simulink model "testbed"  (R2017b)
settings: Solver=FixedStepAuto  StartTime=0.0  StopTime=inf  FixedStep=0.001  RelTol=1e-3  EnableMultiTasking=on
libraries: xpcethercatlib x22, slrtlib x1
settings Model: xpc_rtwmakecfg_data=_xpcethercatlib_  SimulationMode=external  Creator=motor_testbed  LastModifiedBy=motor_testbed
settings SolverCC: ConcurrentTasks=on  AutoInsertRateTranBlk=on
settings DataIOCC: SaveFormat=StructureWithTime
settings OptimizationCC: BlockReduction=off  OptimizeBlockIOStorage=off  BufferReuse=off  GlobalBufferReuse=off  ExpressionFolding=off  LocalBlockOutputs=off
settings HardwareCC: ProdBitPerPointer=32  ProdBitPerSizeT=32  ProdBitPerPtrDiffT=32  ProdLargestAtomicFloat=None  ProdWordSize=32  ProdLongLongMode=on  ProdHWDeviceType=Generic->32-bit x86 compatible
settings RTWCC: SystemTargetFile=slrt.tlc  TemplateMakefile=slrt_default_tmf  Description=Simulink Real-Time  CodeExecutionProfiling=on  RTWCompilerOptimization=on
settings SimulinkRealTimeCC: SupportVariableSizeSignals=on  RL32LogTETModifier=off  xPCConcurrentTasks=on

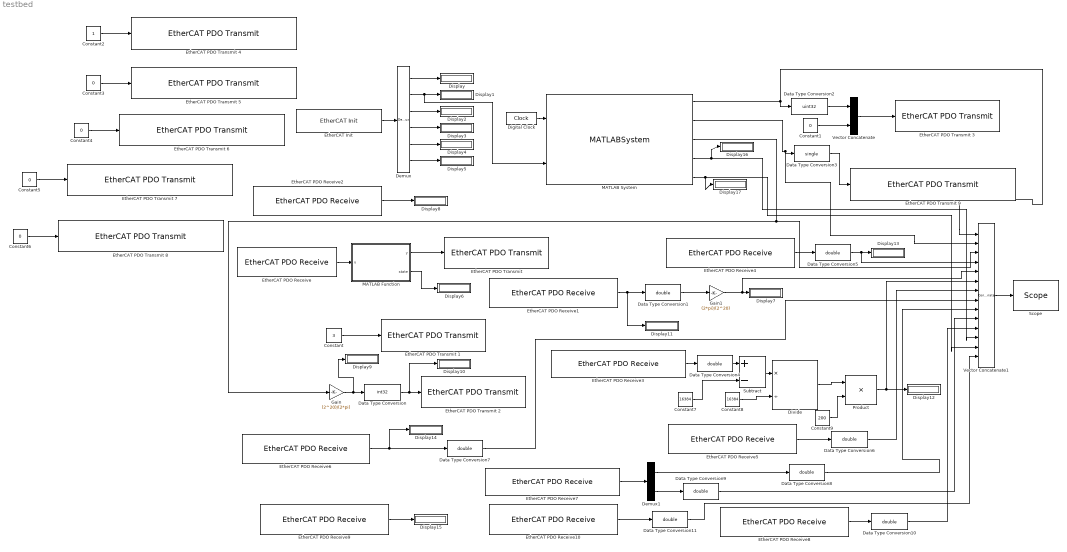
== system testbed ==
  Constant : Constant  Value=3  OutDataTypeStr=int8  SampleTime=0.001
  Constant1 : Constant  Value=0  OutDataTypeStr=uint32  SampleTime=0.001
  Constant2 : Constant  OutDataTypeStr=uint32  SampleTime=0.001
  Constant{3..6} (4 alike) : Constant  Value=0  OutDataTypeStr=single  SampleTime=0.001
  Constant7 : Constant  Value=16384  OutDataTypeStr=double  SampleTime=0.001
  Constant8 : Constant  Value=16384  OutDataTypeStr=double  SampleTime=0.001
  Constant9 : Constant  Value=200  OutDataTypeStr=double  SampleTime=0.001
  Data Type Conversion : DataTypeConversion  OutDataTypeStr=int32
  Data Type Conversion{1,4..11} (9 alike) : DataTypeConversion  OutDataTypeStr=double
  Data Type Conversion2 : DataTypeConversion  OutDataTypeStr=uint32
  Data Type Conversion3 : DataTypeConversion  OutDataTypeStr=single
  Demux : Demux  Outputs=6
  Demux1 : Demux  Outputs=2
  Digital Clock : DigitalClock  SampleTime=0.001
  Display{,1..17} (18 alike) : Display
  Divide : Product  Inputs=*/
  "EtherCAT Init " : xpcethercatlib/EtherCAT Init   Priority=0  config_file=C:\Users\motor_testbed\Desktop\tmotor_testbed\t.xml  device_id=0  pci_bus=5  pci_slot=0  pci_function=0  dctuning=0  enaDebug=off  enaDC=on  errLink=off  masterDbg=off  stateChgDbg=off  baseClock=off  masterCfg=off  logFile='h:\dbglog.txt'  sample_time=0.001000  DCMode=2
      settings: SourceProductName=Simulink Real-Time  SourceProductBaseCode=XP
  EtherCAT PDO Receive : xpcethercatlib/EtherCAT PDO Receive  Priority=2  sig_name=Drive 5 (Elmo Drive ).Inputs.Statusword  sig_offset=1736  sig_type=uint16  type_size=16  sig_dim=1  device_id=0  sample_time=0.001000
      settings: SourceProductName=Simulink Real-Time  SourceProductBaseCode=XP
  EtherCAT PDO Receive1 : xpcethercatlib/EtherCAT PDO Receive  Priority=2  sig_name=Drive 5 (Elmo Drive ).Inputs.Velocity actual value  sig_offset=1760  sig_type=int32  type_size=32  sig_dim=1  device_id=0  sample_time=0.001000
      settings: SourceProductName=Simulink Real-Time  SourceProductBaseCode=XP
  EtherCAT PDO Receive10 : xpcethercatlib/EtherCAT PDO Receive  Priority=2  sig_name=Box 1 (baer_motor_testbed).Inputs.motor_velocity_act  sig_offset=664  sig_type=single  type_size=32  sig_dim=1  device_id=0  sample_time=0.001
      settings: SourceProductName=Simulink Real-Time  SourceProductBaseCode=XP
  EtherCAT PDO Receive2 : xpcethercatlib/EtherCAT PDO Receive  Priority=2  sig_name=Drive 5 (Elmo Drive ).Inputs.Modes of operation display  sig_offset=1752  sig_type=int8  type_size=8  sig_dim=1  device_id=0  sample_time=0.001000
      settings: SourceProductName=Simulink Real-Time  SourceProductBaseCode=XP
  EtherCAT PDO Receive3 : xpcethercatlib/EtherCAT PDO Receive  Priority=2  sig_name=Term 3 (EL3064).AI Standard Channel 4.Value  sig_offset=1624  sig_type=int16  type_size=16  sig_dim=1  device_id=0  sample_time=0.001000
      settings: SourceProductName=Simulink Real-Time  SourceProductBaseCode=XP
  EtherCAT PDO Receive4 : xpcethercatlib/EtherCAT PDO Receive  Priority=2  sig_name=Box 1 (baer_motor_testbed).Inputs.motor_torque_act  sig_offset=696  sig_type=single  type_size=32  sig_dim=1  device_id=0  sample_time=0.001000
      settings: SourceProductName=Simulink Real-Time  SourceProductBaseCode=XP
  EtherCAT PDO Receive5 : xpcethercatlib/EtherCAT PDO Receive  Priority=2  sig_name=Box 1 (baer_motor_testbed).Inputs.motor_status  sig_offset=888  sig_type=uint32  type_size=32  sig_dim=1  device_id=0  sample_time=0.001
      settings: SourceProductName=Simulink Real-Time  SourceProductBaseCode=XP
  EtherCAT PDO Receive6 : xpcethercatlib/EtherCAT PDO Receive  Priority=2  sig_name=Box 1 (baer_motor_testbed).Inputs.can1_error_counter  sig_offset=824  sig_type=uint32  type_size=32  sig_dim=1  device_id=0  sample_time=0.001000
      settings: SourceProductName=Simulink Real-Time  SourceProductBaseCode=XP
  EtherCAT PDO Receive7 : xpcethercatlib/EtherCAT PDO Receive  Priority=2  sig_name=Term 3 (EL3064).AI Standard Channel 4.Status  sig_offset=1608  sig_type=uint8  type_size=8  sig_dim=2  device_id=0  sample_time=0.001000
      settings: SourceProductName=Simulink Real-Time  SourceProductBaseCode=XP
  EtherCAT PDO Receive8 : xpcethercatlib/EtherCAT PDO Receive  Priority=2  sig_name=Drive 5 (Elmo Drive ).Inputs.Torque actual value  sig_offset=1824  sig_type=int16  type_size=16  sig_dim=1  device_id=0  sample_time=0.001000
      settings: SourceProductName=Simulink Real-Time  SourceProductBaseCode=XP
  EtherCAT PDO Receive9 : xpcethercatlib/EtherCAT PDO Receive  Priority=2  sig_name=Drive 5 (Elmo Drive ).Inputs.Modes of operation display  sig_offset=1752  sig_type=int8  type_size=8  sig_dim=1  device_id=0  sample_time=0.001000
      settings: SourceProductName=Simulink Real-Time  SourceProductBaseCode=XP
  "EtherCAT PDO Transmit " : xpcethercatlib/EtherCAT PDO Transmit   Priority=3  sig_name=Drive 5 (Elmo Drive ).Outputs.Controlword  sig_offset=1736  sig_type=uint16  type_size=16  sig_dim=1  device_id=0  sample_time=0.001000
      settings: SourceProductName=Simulink Real-Time  SourceProductBaseCode=XP
  EtherCAT PDO Transmit 1 : xpcethercatlib/EtherCAT PDO Transmit   Priority=3  sig_name=Drive 5 (Elmo Drive ).Outputs.Modes of operation  sig_offset=1784  sig_type=int8  type_size=8  sig_dim=1  device_id=0  sample_time=0.001000
      settings: SourceProductName=Simulink Real-Time  SourceProductBaseCode=XP
  EtherCAT PDO Transmit 2 : xpcethercatlib/EtherCAT PDO Transmit   Priority=3  sig_name=Drive 5 (Elmo Drive ).Outputs.Target velocity  sig_offset=1752  sig_type=int32  type_size=32  sig_dim=1  device_id=0  sample_time=0.001000
      settings: SourceProductName=Simulink Real-Time  SourceProductBaseCode=XP
  EtherCAT PDO Transmit 3 : xpcethercatlib/EtherCAT PDO Transmit   Priority=3  sig_name=Box 1 (baer_motor_testbed).Outputs.hs  sig_offset=568  sig_type=uint32  type_size=32  sig_dim=2  device_id=0  sample_time=0.001000
      settings: SourceProductName=Simulink Real-Time  SourceProductBaseCode=XP
  EtherCAT PDO Transmit 4 : xpcethercatlib/EtherCAT PDO Transmit   Priority=3  sig_name=Box 1 (baer_motor_testbed).Outputs.control_word  sig_offset=824  sig_type=uint32  type_size=32  sig_dim=1  device_id=0  sample_time=0.001000
      settings: SourceProductName=Simulink Real-Time  SourceProductBaseCode=XP
  EtherCAT PDO Transmit 5 : xpcethercatlib/EtherCAT PDO Transmit   Priority=3  sig_name=Box 1 (baer_motor_testbed).Outputs.motor_position_des  sig_offset=632  sig_type=single  type_size=32  sig_dim=1  device_id=0  sample_time=0.001000
      settings: SourceProductName=Simulink Real-Time  SourceProductBaseCode=XP
  EtherCAT PDO Transmit 6 : xpcethercatlib/EtherCAT PDO Transmit   Priority=3  sig_name=Box 1 (baer_motor_testbed).Outputs.motor_velocity_des  sig_offset=664  sig_type=single  type_size=32  sig_dim=1  device_id=0  sample_time=0.001000
      settings: SourceProductName=Simulink Real-Time  SourceProductBaseCode=XP
  EtherCAT PDO Transmit 7 : xpcethercatlib/EtherCAT PDO Transmit   Priority=3  sig_name=Box 1 (baer_motor_testbed).Outputs.motor_kp  sig_offset=728  sig_type=single  type_size=32  sig_dim=1  device_id=0  sample_time=0.001000
      settings: SourceProductName=Simulink Real-Time  SourceProductBaseCode=XP
  EtherCAT PDO Transmit 8 : xpcethercatlib/EtherCAT PDO Transmit   Priority=3  sig_name=Box 1 (baer_motor_testbed).Outputs.motor_kd  sig_offset=760  sig_type=single  type_size=32  sig_dim=1  device_id=0  sample_time=0.001000
      settings: SourceProductName=Simulink Real-Time  SourceProductBaseCode=XP
  EtherCAT PDO Transmit 9 : xpcethercatlib/EtherCAT PDO Transmit   Priority=3  sig_name=Box 1 (baer_motor_testbed).Outputs.motor_torque_des  sig_offset=696  sig_type=single  type_size=32  sig_dim=1  device_id=0  sample_time=0.001000
      settings: SourceProductName=Simulink Real-Time  SourceProductBaseCode=XP
  Gain : Gain  Gain=(2^20)/(2*pi)
  Gain1 : Gain  Gain=(2*pi)/(2^20)
  MATLAB Function : MATLAB Function  TreatAsAtomicUnit=on
  MATLAB System : MATLABSystem  System=InfoS  SimulateUsing=Code generation
      mask Type: InfoS
      mask Display:
      | disp('InfoS');
      | port_label('input',1,'t');
      | port_label('input',2,'ecat_status');
      | port_label('output',1,'hss');
      | port_label('output',2,'motor_torque');
      | port_label('output',3,'load_speed');
      | port_label('output',4,'speed_state');
      | port_label('output',5,'torque_state');
  Product : Product
  "Scope " : slrtlib/Displays and Logging/Scope   scopeno=1  scopetype=File  autostart=on  viewmode=Graphical redraw  formatstr='%15.6f'  grid=on  ylimits=[0,0]  nosamples=1000  noprepostsamples=0  interleave=1  triggermode=FreeRun  triggersignal=1  trigsignalfromport=off  triggerlevel=0.0  triggerslope=Either  triggerscope=1  triggersample=0  filename=cadata.dat  mode=Commit  writesize=1024  autorestart=on  dynamicfilemode=off  maxwritefilesize=2*1024*1024^2
  Subtract : Sum  Inputs=+-
  Vector Concatenate : Concatenate
  Vector Concatenate1 : Concatenate  NumInputs=14
  wires:
  "EtherCAT Init "/1 -> Demux/1
  Demux/1 -> Display/1
  Demux/2 -> MATLAB System/2, Display1/1
  Demux/3 -> Display2/1
  Demux/4 -> Display3/1
  Demux/5 -> Display4/1
  Demux/6 -> Display5/1
  EtherCAT PDO Receive/1 -> MATLAB Function/1(u)
  MATLAB Function/1(y) -> "EtherCAT PDO Transmit "/1
  MATLAB Function/2(state) -> Display6/1
  Constant/1 -> EtherCAT PDO Transmit 1/1
  Gain1/1 -> Vector Concatenate1/5, Display7/1
  Gain/1 -> Display9/1, Data Type Conversion/1
  Data Type Conversion/1 -> Display10/1, EtherCAT PDO Transmit 2/1
  Data Type Conversion1/1 -> Gain1/1
  EtherCAT PDO Receive1/1 -> Display11/1, Data Type Conversion1/1
  EtherCAT PDO Receive2/1 -> Display8/1
  MATLAB System/3 -> Vector Concatenate1/3, Gain/1
  Digital Clock/1 -> MATLAB System/1
  Vector Concatenate/1 -> EtherCAT PDO Transmit 3/1
  MATLAB System/1 -> Vector Concatenate1/1, Data Type Conversion2/1
  Data Type Conversion2/1 -> Vector Concatenate/1
  Constant1/1 -> Vector Concatenate/2
  Constant2/1 -> EtherCAT PDO Transmit 4/1
  Constant3/1 -> EtherCAT PDO Transmit 5/1
  Constant4/1 -> EtherCAT PDO Transmit 6/1
  Constant5/1 -> EtherCAT PDO Transmit 7/1
  Constant6/1 -> EtherCAT PDO Transmit 8/1
  MATLAB System/2 -> Vector Concatenate1/2, Data Type Conversion3/1
  Data Type Conversion3/1 -> EtherCAT PDO Transmit 9/1
  Constant7/1 -> Subtract/2
  Subtract/1 -> Divide/1
  Constant8/1 -> Divide/2
  Divide/1 -> Product/1
  Constant9/1 -> Product/2
  Product/1 -> Vector Concatenate1/6, Display12/1
  EtherCAT PDO Receive3/1 -> Data Type Conversion4/1
  Data Type Conversion4/1 -> Subtract/1
  EtherCAT PDO Receive4/1 -> Data Type Conversion5/1
  Data Type Conversion5/1 -> Vector Concatenate1/4, Display13/1
  Vector Concatenate1/1 -> "Scope "/1
  EtherCAT PDO Receive5/1 -> Data Type Conversion6/1
  Data Type Conversion6/1 -> Vector Concatenate1/7
  EtherCAT PDO Receive6/1 -> Data Type Conversion7/1, Display14/1
  Data Type Conversion7/1 -> Vector Concatenate1/8
  Data Type Conversion8/1 -> Vector Concatenate1/9
  EtherCAT PDO Receive7/1 -> Demux1/1
  Demux1/2 -> Data Type Conversion9/1
  Demux1/1 -> Data Type Conversion8/1
  Data Type Conversion9/1 -> Vector Concatenate1/10
  EtherCAT PDO Receive8/1 -> Data Type Conversion10/1
  Data Type Conversion10/1 -> Vector Concatenate1/11
  EtherCAT PDO Receive9/1 -> Display15/1
  MATLAB System/4 -> Display16/1, Vector Concatenate1/12
  MATLAB System/5 -> Display17/1, Vector Concatenate1/13
  EtherCAT PDO Receive10/1 -> Data Type Conversion11/1
  Data Type Conversion11/1 -> Vector Concatenate1/14

== matlab function testbed/MATLAB Function ==
  data: u input; y output; state output
function [y, state] = state_machine(u)

    persistent state_code current_state sub_state
    if isempty(state_code)
        state_code = 0;
        current_state = 0;
        sub_state = 0;
    end
    
    if bitand(u, uint16(hex2dec('6F'))) == hex2dec('27')
        state_code = 5; % Operation enabled
    elseif bitand(u, uint16(hex2dec('4F'))) == hex2dec('f')
        state_code = -2; % Fault reaction active
    elseif bitand(u, uint16(hex2dec('4F'))) == hex2dec('40')
        state_code = 2; % Switch on disabled   
    elseif bitand(u, uint16(hex2dec('4F'))) == 8
        state_code = -3; % fault
    elseif bitand(u, uint16(hex2dec('4F'))) == 0
        state_code = 1; % not ready to switch on
    elseif bitand(u, uint16(hex2dec('6F'))) == hex2dec('21')
        state_code = 3; %Ready to switch on
    elseif bitand(u, uint16(hex2dec('6F'))) == hex2dec('23')
        state_code = 4; % Switch on
    elseif bitand(u, uint16(hex2dec('6F'))) == hex2dec('07')
        state_code = -1; % Quick stop active
    end
    
    y = uint16(hex2dec('0'));
    state = current_state;
    if state_code > 1
        if current_state == 0 % for fault reset
            y = uint16(hex2dec('80'));
            sub_state = sub_state + 1;
            if sub_state == 11
                current_state = 1;
                sub_state = 0;
            end
        elseif current_state == 1 % for shutdown
            y = uint16(hex2dec('6'));
            sub_state = sub_state + 1;
            if sub_state == 11
                current_state = 2;
                sub_state = 0;
            end
        elseif current_state == 2 % for SwitchON
            y = uint16(hex2dec('7'));
            sub_state = sub_state + 1;
            if sub_state == 11
                current_state = 3;
                sub_state = 0;
            end
        elseif current_state == 3 % for operationEn
            y = uint16(hex2dec('f'));
            sub_state = sub_state + 1;
            if sub_state == 11
                current_state = 4;
                sub_state = 0;
            end
         elseif current_state == 4 % for operationEn
            y = uint16(hex2dec('f'));
        end
    else
        state = state_code;
    end
end
